simulink model "untitled"  (R2022b)
settings: Solver=VariableStepAuto  StartTime=0.0  StopTime=35  RelTol=1e-3
libraries: simulink_extras x1
settings Model: Creator=sohamkarak  LastModifiedBy=sohamkarak

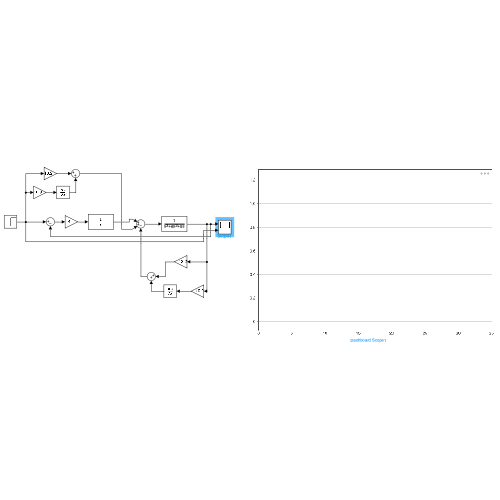
[thumbnail: Simulink's stored preview of the top-level diagram]
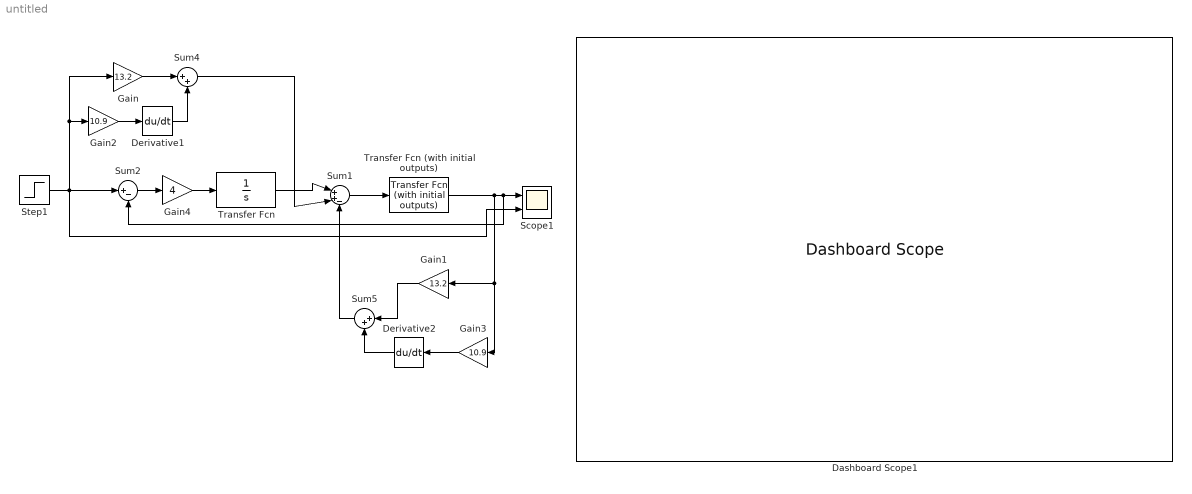
== system untitled ==
  Dashboard Scope1 : DashboardScope
  Derivative1 : Derivative
  Derivative2 : Derivative
  Gain : Gain  Gain=13.2
  Gain1 : Gain  Gain=13.2
  Gain2 : Gain  Gain=10.9
  Gain3 : Gain  Gain=10.9
  Gain4 : Gain  Gain=4
  Scope1 : Scope  NumInputPorts=2
  Step1 : Step  SampleTime=0
  Sum1 : Sum  Inputs=|++-
  Sum2 : Sum  Inputs=|+-
  Sum4 : Sum  Inputs=|++
  Sum5 : Sum  Inputs=|++
  Transfer Fcn : TransferFcn  Denominator=[1 0]
  Transfer Fcn (with initial outputs) : simulink_extras/Additional Linear/Transfer Fcn (with initial outputs)  N=[1]  D=[1 6 5 0]  Y0=0  U0=0
  wires:
  Transfer Fcn/1 -> Sum1/1
  Sum1/1 -> Transfer Fcn (with initial outputs)/1
  Sum4/1 -> Sum1/2
  Gain/1 -> Sum4/1
  Derivative1/1 -> Sum4/2
  Gain1/1 -> Sum5/1
  Step1/1 -> Scope1/2, Sum2/1, Gain/1, Gain2/1
  Transfer Fcn (with initial outputs)/1 -> Sum2/2, Scope1/1, Gain3/1, Gain1/1
  Sum5/1 -> Sum1/3
  Derivative2/1 -> Sum5/2
  Gain2/1 -> Derivative1/1
  Gain3/1 -> Derivative2/1
  Sum2/1 -> Gain4/1
  Gain4/1 -> Transfer Fcn/1
